simulink model "sf_change_detection_vector"  (Simulink 7.6)
settings: Solver=FixedStepDiscrete  StartTime=0.0  StopTime=10.0  FixedStep=1  RelTol=1e-3
libraries: simulink x1
settings Model: Creator=The MathWorks Inc.  ExtModeAutoUpdateStatusClock=off
settings OptimizationCC: InitFltsAndDblsToZero=on  EfficientMapNaN2IntZero=off
settings DebuggingCC: SolverPrmCheckMsg=none  StrictBusMsg=Warning
settings SFSimCC: SimParseCustomCode=off

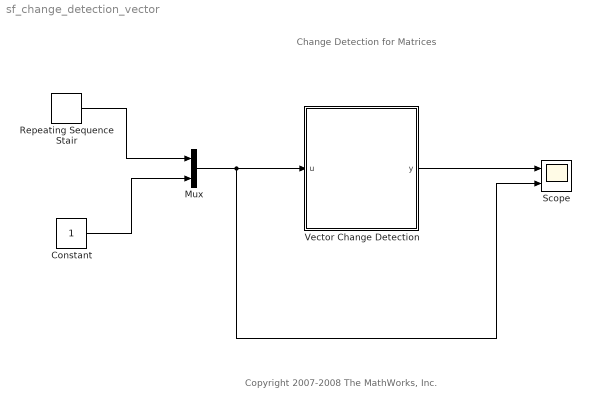
== system sf_change_detection_vector ==
  note: Change Detection for Matrices
  note: Copyright 2007-2008 The MathWorks, Inc.
  Constant : Constant
  Mux : Mux  Inputs=2
  Repeating Sequence Stair : simulink/Sources/Repeating Sequence Stair  SystemSampleTime=-1  OutValues=[1 2 3]  tsamp=-1  OutMin=[]  OutMax=[]  OutDataTypeStr=float('double')  OutputDataTypeScalingMode=Specify via dialog  OutDataType=float('double')  ConRadixGroup=Best Precision: Vector-wise  OutScaling=2^-12
  Scope : Scope  NumInputPorts=2
      settings: YMin=-5~-5  YMax=5~5
  Vector Change Detection : Stateflow chart  TreatAsAtomicUnit=on
  wires:
  Constant/1 -> Mux/2
  Mux/1 -> Vector Change Detection/1(u), Scope/2
  Vector Change Detection/1(y) -> Scope/1
  Repeating Sequence Stair/1 -> Mux/1

== stateflow chart Vector Change Detection ==
  state S
    en: y += hasChanged(u);
  (default) -> S
  S -> S
  data: u input double; y output double
